simulink model "WaveletDenoising"  (Simulink 6.5)
settings: Solver=FixedStepDiscrete  SolverMode=SingleTasking  StartTime=0.0  StopTime=1024  RelTol=1e-3
model workspace: external: MAT-File (data not in the file)
undefined symbols (not defined in the file or in its folder): lod, ts
libraries: dspmlti4 x6, dspsigops x3, dspmisc x1, dspsrcs4 x1
settings Model: Creator=The MathWorks Inc.  LastModifiedBy=Administrator  ExtModeTrigMode=oneshot  ExtModeArmWhenConnect=off  ExtModeAutoUpdateStatusClock=off
settings DataIOCC: LimitDataPoints=off  SaveOutput=off  SaveTime=off  SignalLoggingName=logsOut
settings OptimizationCC: BlockReduction=off  BooleanDataType=off  InlineInvariantSignals=on
settings DebuggingCC: SolverPrmCheckMsg=none  MultiTaskDSMMsg=warning  MultiTaskCondExecSysMsg=none  IntegerOverflowMsg=none  StrictBusMsg=None
settings HardwareCC: TargetUnknown=on
settings RTWCC: IncludeERTFirstTime=on

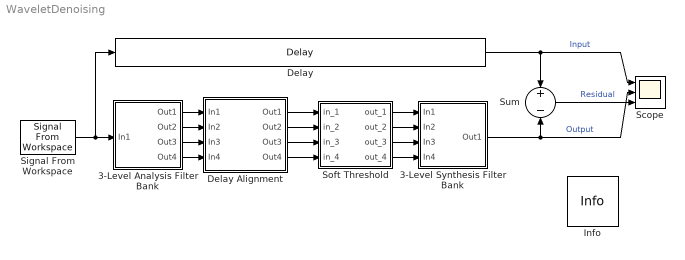
== system WaveletDenoising ==
  3-Level Analysis Filter Bank : Subsystem
  3-Level Synthesis Filter Bank : Subsystem
  Delay : dspsigops/Delay  dly_unit=Samples  delay=7*(length(lod)-1)  ic_detail=on  dif_ic_for_ch=off  dif_ic_for_dly=off  ic=0  reset_popup=None
  Delay Alignment : Subsystem
  Info : dspmisc/Info  SystemSampleTime=-1
  Scope : Scope  NumInputPorts=3
      settings: TimeRange=1025  YMin=-10~-10~-5  YMax=10~10~5
  Signal From Workspace : dspsrcs4/Signal From Workspace  SystemSampleTime=-1  X=noisdopp  Ts=ts  nsamps=1  OutputAfterFinalValue=Setting to zero  ignoreOrWarnInputAndFrameLengths=off
  Soft Threshold : Subsystem  mask(Soft Threshold){st=[3 2 1 0]}
      mask prompts: st "Vector of thresholds for each level:"
      mask help: Apply a soft threshold (deadzone transfer function) to each signal in the decomposition. First threshold applies to top-most filter bank output.
      mask init:
      | x=([-1 1 NaN 0 0 NaN -1 -.5 .5 1]+1)/2*.7+.15;
      | y=([0 0 NaN -1 1 NaN -1 0 0 1]+1)/2*.7+.05;
      mask Help: Vector of thresholds for each decomposition level.
      mask Display:
      | text(.1,.9,'Dead Zone')
      | plot(x,y)
  Sum : Sum  Inputs=+-  SaturateOnIntegerOverflow=on  InputSameDT=on
  wires:
  Signal From Workspace/1 -> 3-Level Analysis Filter Bank/1(In1), Delay/1
  Soft Threshold/1(out_1) -> 3-Level Synthesis Filter Bank/1(In1)
  Soft Threshold/2(out_2) -> 3-Level Synthesis Filter Bank/2(In2)
  Soft Threshold/3(out_3) -> 3-Level Synthesis Filter Bank/3(In3)
  Soft Threshold/4(out_4) -> 3-Level Synthesis Filter Bank/4(In4)
  Delay/1 -> Sum/1, Scope/1  "Input"
  3-Level Synthesis Filter Bank/1(Out1) -> Sum/2, Scope/2  "Output"
  Sum/1 -> Scope/3  "Residual"
  3-Level Analysis Filter Bank/1(Out1) -> Delay Alignment/1(In1)
  3-Level Analysis Filter Bank/2(Out2) -> Delay Alignment/2(In2)
  3-Level Analysis Filter Bank/3(Out3) -> Delay Alignment/3(In3)
  3-Level Analysis Filter Bank/4(Out4) -> Delay Alignment/4(In4)
  Delay Alignment/1(Out1) -> Soft Threshold/1(in_1)
  Delay Alignment/2(Out2) -> Soft Threshold/2(in_2)
  Delay Alignment/3(Out3) -> Soft Threshold/3(in_3)
  Delay Alignment/4(Out4) -> Soft Threshold/4(in_4)

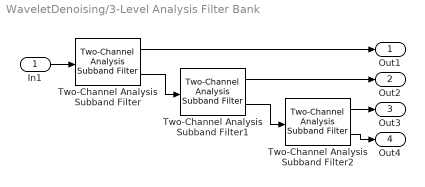
== system WaveletDenoising/3-Level Analysis Filter Bank ==
  In1 : Inport
  Two-Channel Analysis Subband Filter : dspmlti4/Two-Channel Analysis Subband Filter  DialogController=dspDDGCreate  DialogControllerArgs=DataTag0  SystemSampleTime=-1  lpf=lod  hpf=hid  framing=Maintain input frame size  roundingMode=Floor  overflowMode=off
  Two-Channel Analysis Subband Filter1 : dspmlti4/Two-Channel Analysis Subband Filter  DialogController=dspDDGCreate  DialogControllerArgs=DataTag1  SystemSampleTime=-1  lpf=lod  hpf=hid  framing=Maintain input frame size  roundingMode=Floor  overflowMode=off
  Two-Channel Analysis Subband Filter2 : dspmlti4/Two-Channel Analysis Subband Filter  DialogController=dspDDGCreate  DialogControllerArgs=DataTag2  SystemSampleTime=-1  lpf=lod  hpf=hid  framing=Maintain input frame size  roundingMode=Floor  overflowMode=off
  Out1 : Outport
  Out2 : Outport  Port=2
  Out3 : Outport  Port=3
  Out4 : Outport  Port=4
  wires:
  Two-Channel Analysis Subband Filter2/2 -> Out4/1
  Two-Channel Analysis Subband Filter2/1 -> Out3/1
  Two-Channel Analysis Subband Filter1/1 -> Out2/1
  In1/1 -> Two-Channel Analysis Subband Filter/1
  Two-Channel Analysis Subband Filter/1 -> Out1/1
  Two-Channel Analysis Subband Filter1/2 -> Two-Channel Analysis Subband Filter2/1
  Two-Channel Analysis Subband Filter/2 -> Two-Channel Analysis Subband Filter1/1

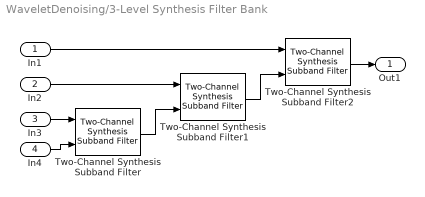
== system WaveletDenoising/3-Level Synthesis Filter Bank ==
  In1 : Inport
  In2 : Inport  Port=2
  In3 : Inport  Port=3
  In4 : Inport  Port=4
  Two-Channel Synthesis Subband Filter : dspmlti4/Two-Channel Synthesis Subband Filter  DialogController=dspDDGCreate  DialogControllerArgs=DataTag3  SystemSampleTime=-1  lpf=lor  hpf=hir  framing=Maintain input frame size  roundingMode=Floor  overflowMode=off
  Two-Channel Synthesis Subband Filter1 : dspmlti4/Two-Channel Synthesis Subband Filter  DialogController=dspDDGCreate  DialogControllerArgs=DataTag4  SystemSampleTime=-1  lpf=lor  hpf=hir  framing=Maintain input frame size  roundingMode=Floor  overflowMode=off
  Two-Channel Synthesis Subband Filter2 : dspmlti4/Two-Channel Synthesis Subband Filter  DialogController=dspDDGCreate  DialogControllerArgs=DataTag5  SystemSampleTime=-1  lpf=lor  hpf=hir  framing=Maintain input frame size  roundingMode=Floor  overflowMode=off
  Out1 : Outport
  wires:
  In4/1 -> Two-Channel Synthesis Subband Filter/2
  In3/1 -> Two-Channel Synthesis Subband Filter/1
  In2/1 -> Two-Channel Synthesis Subband Filter1/1
  Two-Channel Synthesis Subband Filter2/1 -> Out1/1
  In1/1 -> Two-Channel Synthesis Subband Filter2/1
  Two-Channel Synthesis Subband Filter1/1 -> Two-Channel Synthesis Subband Filter2/2
  Two-Channel Synthesis Subband Filter/1 -> Two-Channel Synthesis Subband Filter1/2

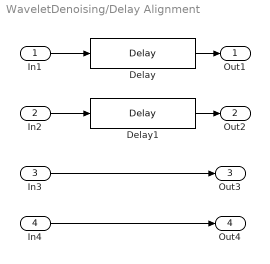
== system WaveletDenoising/Delay Alignment ==
  In1 : Inport
  In2 : Inport  Port=2
  In3 : Inport  Port=3
  In4 : Inport  Port=4
  Delay : dspsigops/Delay  dly_unit=Samples  delay=3*(length(lod)-1)  ic_detail=on  dif_ic_for_ch=off  dif_ic_for_dly=off  ic=0  reset_popup=None
  Delay1 : dspsigops/Delay  dly_unit=Samples  delay=length(lod) - 1  ic_detail=on  dif_ic_for_ch=off  dif_ic_for_dly=off  ic=0  reset_popup=None
  Out1 : Outport
  Out2 : Outport  Port=2
  Out3 : Outport  Port=3
  Out4 : Outport  Port=4
  wires:
  In3/1 -> Out3/1
  In4/1 -> Out4/1
  In2/1 -> Delay1/1
  Delay1/1 -> Out2/1
  In1/1 -> Delay/1
  Delay/1 -> Out1/1

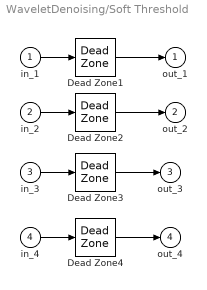
== system WaveletDenoising/Soft Threshold ==
  in_1 : Inport
  in_2 : Inport  Port=2
  in_3 : Inport  Port=3
  in_4 : Inport  Port=4
  Dead Zone1 : DeadZone  LowerValue=-st(1)  UpperValue=st(1)  ZeroCross=off  SaturateOnIntegerOverflow=on
  Dead Zone2 : DeadZone  LowerValue=-st(2)  UpperValue=st(2)  ZeroCross=off  SaturateOnIntegerOverflow=on
  Dead Zone3 : DeadZone  LowerValue=-st(3)  UpperValue=st(3)  ZeroCross=off  SaturateOnIntegerOverflow=on
  Dead Zone4 : DeadZone  LowerValue=-st(4)  UpperValue=st(4)  ZeroCross=off  SaturateOnIntegerOverflow=on
  out_1 : Outport  InitialOutput=0
  out_2 : Outport  Port=2  InitialOutput=0
  out_3 : Outport  Port=3  InitialOutput=0
  out_4 : Outport  Port=4  InitialOutput=0
  wires:
  in_1/1 -> Dead Zone1/1
  Dead Zone1/1 -> out_1/1
  in_2/1 -> Dead Zone2/1
  Dead Zone2/1 -> out_2/1
  in_3/1 -> Dead Zone3/1
  Dead Zone3/1 -> out_3/1
  in_4/1 -> Dead Zone4/1
  Dead Zone4/1 -> out_4/1
